simulink model "Control_test"  (R2014b)
settings: Solver=FixedStepDiscrete  StartTime=0.0  StopTime=Inf  FixedStep=0.001  RelTol=1e-3
PostLoadFcn:
  | , if any(exist('dsrtsu_mdlpostloadfcn', 'file') == [2, 3, 6]), try dsrtsu_mdlpostloadfcn('Execute', bdroot); catch fprintf('Error in PostLoadFcn (dsrtsu_mdlpostloadfcn) for model "%s":\n %s\n', bdroot, lasterr); end, end,
undefined symbols (not defined in the file or in its folder): dtLocal, slcm
libraries: rtican x163, simulink x14
(part 14 of 34)

== system Control_test/InputProcessing/RadarCanProcessing/ESR_Sim1 ==
  Bus Creator : BusCreator  Inputs=9
  ESR_Sim1 : rtican/RTICAN Receive (RX)   Reserved1=[]  Reserved2=[]  Reserved3=[]  Reserved4=[]  SfcnMessage=[]  Msg_Struct=[]  BoardTypeNo=[]  BoardNo=[]  ChannelNo=[]  Parameters=[]  DialogFcn=[]  UnitName=[]  Revision=[]  UnitValues=[]  DSProperties=struct('RTI',struct('Version',uint32(5),'BlockType',struct('isSLSource',uint8(1),'isSLSink',uint8(1),'isHWSource',uint8(0),'isHWSink',uint8(0),'isSetup',uint8(0),'isInline',uint8(1),'isNonInline',uint8(0),'isInterrupt',uint8(0),'isChannelwise',uint8(0)),'IOBoardType','RTICAN','UnitType','MESSAGE','Identifier','RX','DialogType','MSVC','BlockSet','RTICAN','SlaveProcessor','CAN'))  RTIBlockInterface=struct('OutputPortsWidth',int32([1 1 1 1 1 1 1 1 1]),'OutputPortsActive',[1 1 1 1 1 1 1 1 1],'OutputPortsName',{{'CAN_RX_SIM_RANGE_RATE','CAN_RX_SIM_RANGE_ACCEL','CAN_RX_SIM_RANGE','CAN_RX_SIM_LAT_RATE','CAN_RX_SIM_LAT_POS','CAN_RX_SIM_ANGLE','CAN_RX_SIM_FUNCTION','CAN_RX_SIM_STATUS','CAN_RX_SIM_TRACK_ID'}},'OutputPortsDataType',{{'SS_DOUBLE','SS_DOUBLE','SS_DOUBLE','SS_DOUBLE','SS_DOUBLE','SS_DOUBLE','SS_DOUBLE','SS_DOUBLE','SS_DOUBLE'}},'OutputPortsLabel',{{'CAN_RX_SIM_RANGE_RATE','CAN_RX_SIM_RANGE_ACCEL','CAN_RX_SIM_RANGE','CAN_RX_SIM_LAT_RATE','CAN_RX_SIM_LAT_POS','CAN_RX_SIM_ANGLE','CAN_RX_SIM_FUNCTION','CAN_RX_SIM_STATUS','CAN_RX_SIM_TRACK_ID'}},'OutputPortsLabelMode','ON','InputPortsWidth',int32(0),'InputPortsActive',0,'DialogFcn','rtican_message_interface_gui','BlockDisplay',{{'','center'}},'IconTransparency','on','ParameterTunableNames',{{}},'InitLevel',3,'BlockName',struct('Token',{{'ESR_Sim1'}}),'SampleTime',{{-1}},'TriggerPort',{{'none'}},'EnablePort',{{'none'}})  RTIBlockParameters=struct('BoardTypeNo',{{1,'OFF',[]}},'BoardNo',{{2,'ON',[1 16]}},'ChannelNo',{{2,'ON',[1 2]}},'Parameters',{{struct('DataFileSupport',struct('DataFileSelectedMaster',1,'DataFileSelectedLocal',1,'DataFileName','c:\users\mpc_car\documents\github\mpc-car\controller\dbcfiles\esr_dv3_64tgt.dbc|','DataFileDate',['26-Aug-2014 13:16:21'],'SelectedFile','..\..\dbcfiles\esr_dv3_64tgt.dbc','InterfaceFcn','rtican_dbc_file_parser'),'Options',struct('StatusSelected',0,'TimeSelected',0,'DeltaTimeSelected',0,'BytePortSelected',0,'MessageLengthSelected',0,'TriggerPort',struct('Selected',0,'TriggerType',0),'UserCoding',struct('Selected',0,'InterfaceFile','UserDecodingFile','FcnName','UserDecodeFcn','InportSelected',0,'InportWidth',1,'OutportSelected',0,'OutportWidth',1),'EnablePortSelected',0,'SignalOnPortnameSelected',1,'UseRXService',0),'Message',struct('MsgOnBlocknameSelected',1,'MsgName','ESR_Sim1','MsgIdFormat',0,'MsgId',1472,'MsgLength',8,'NumSignals',9,'SampleTime',-1,'Signal',struct('SgnName',{'CAN_RX_SIM_RANGE_RATE','CAN_RX_SIM_RANGE_ACCEL','CAN_RX_SIM_RANGE','CAN_RX_SIM_LAT_RATE','CAN_RX_SIM_LAT_POS','CAN_RX_SIM_ANGLE','CAN_RX_SIM_FUNCTION','CAN_RX_SIM_STATUS','CAN_RX_SIM_TRACK_ID'},'SgnStartBit',{8,16,24,32,40,48,56,59,61},'SgnLength',{8,8,8,8,8,8,3,2,2},'ByteLayout',{2,2,2,2,2,2,2,2,2},'Factor',{0.25,0.25,1,0.25,0.25,0.5,1,1,1},'Offset',{0,0,0,0,0,0,0,0,0},'SgnComment',{'','','','','','','','',''},'SgnUnit',{'m/s','m/s/s','m','m/s','m','deg','','',''},'Min',{-32,-32,0,-32,-32,-64,0,0,0},'Max',{31.75,31.75,0,31.75,31.75,63.5,0,0,0},'SgnType',{0,0,0,0,0,0,0,0,0},'SLDataType',{'SS_DOUBLE','SS_DOUBLE','SS_DOUBLE','SS_DOUBLE','SS_DOUBLE','SS_DOUBLE','SS_DOUBLE','SS_DOUBLE','SS_DOUBLE'},'DataType',{1,1,0,1,1,1,0,0,0},'ModeValue',{-1,-1,-1,-1,-1,-1,-1,-1,-1}),'MsgIdNumFormat',0,'MsgComment',{{''}}),'Version',1.2,'general',struct('isFromLib',0)),'OFF',[]}},'GroupId',{{struct('Group',{{'RTICAN'}},'No',4,'Behavior',{{'NAMECHANGE'}},'BlockType',{{'SINK'}},'NameChangeFlag',0),'OFF',[]}},'SFcnRTICANMessage',{{struct('MsgType','RX','SFcnPortType','Scalar','MsgName','ESR_Sim1','MsgIdFormat','STD','MsgId',1472,'MsgLength',8,'NumSignals',9,'SampleTime',-1,'Signal',struct('SgnName',{'CAN_RX_SIM_RANGE_RATE','CAN_RX_SIM_RANGE_ACCEL','CAN_RX_SIM_RANGE','CAN_RX_SIM_LAT_RATE','CAN_RX_SIM_LAT_POS','CAN_RX_SIM_ANGLE','CAN_RX_SIM_FUNCTION','CAN_RX_SIM_STATUS','CAN_RX_SIM_TRACK_ID'},'SgnStartBit',{8,16,24,32,40,48,56,59,61},'SgnLength',{8,8,8,8,8,8,3,2,2},'ByteLayout',{['motorola back.'],['motorola back.'],['motorola back.'],['motorola back.'],['motorola back.'],['motorola back.'],['motorola back.'],['motorola back.'],['motorola back.']},'Factor',{0.25,0.25,1,0.25,0.25,0.5,1,1,1},'Offset',{0,0,0,0,0,0,0,0,0},'SgnType',{'standard','standard','standard','standard','standard','standard','standard','standard','standard'},'SLDataType',{'SS_DOUBLE','SS_DOUBLE','SS_DOUBLE','SS_DOUBLE','SS_DOUBLE','SS_DOUBLE','SS_DOUBLE','SS_DOUBLE','SS_DOUBLE'},'DataType',{['signed int'],['signed int'],['unsigned int'],['signed int'],['signed int'],['signed int'],['unsigned int'],['unsigned int'],['unsigned int']},'ModeValue',{-1,-1,-1,-1,-1,-1,-1,-1,-1}),'StatusSelected','no','TimeSelected','no','DeltaTimeSelected','no','BytePortSelected','no','MessageLengthSelected','no','TriggerPort',struct('Selected','no','TriggerType',0),'UserCoding',struct('Selected','no','InterfaceFile','UserDecodingFile','FcnName','UserDecodeFcn','InportSelected','no','InportWidth',1,'OutportSelected','no','OutportWidth',1),'EnablePortSelected','no','UseRXService','no','BoardType','DS1','BoardNo',2,'ControllerNo',2),'OFF',[]}},'TLCFileName',{{'rtican_rx_message','OFF',[]}})  RTISFcnParameters=struct('SFcnRTICANMessage','struct','TLCFileName','char')  RTIBlockParaDefault=struct('BoardTypeNo',4302,'BoardNo',1,'ChannelNo',1,'Parameters',struct('DataFileSupport',struct('DataFileSelectedMaster',0,'DataFileSelectedLocal',0,'DataFileName','','DataFileDate','','SelectedFile',['<no file selected>']),'Options',struct('StatusSelected',1,'TimeSelected',1,'DeltaTimeSelected',1,'BytePortSelected',0,'MessageLengthSelected',0,'TriggerPort',struct('Selected',0,'TriggerType','rising'),'UserCoding',struct('Selected',0,'InterfaceFile','UserDecodingFile','FcnName','UserDecodeFcn','InportSelected',0,'InportWidth',1,'OutportSelected',0,'OutportWidth',1),'EnablePortSelected',0,'SignalOnPortnameSelected',1,'UseRXService',0),'Message',struct('MsgOnBlocknameSelected',0,'MsgName',['RX Message'],'MsgIdFormat',0,'MsgId',100,'MsgLength',8,'NumSignals',1,'SampleTime',-1,'Signal',struct('SgnName',['RX signal'],'SgnStartBit',0,'SgnLength',8,'SgnType',0,'ModeValue',-1,'DataType',0,'SLDataType','SS_DOUBLE','ByteLayout',0,'Factor',1,'Offset',0,'Min',0,'Max',255,'SgnComment',{{}},'SgnUnit',''),'MsgIdNumFormat',0,'MsgComment',{{''}}),'Version',1.2,'general',struct('isFromLib',1)),'GroupId',struct('Group',{{'RTICAN'}},'No',1,'Behavior',{{'NAMECHANGE'}},'BlockType',{{'SINK'}},'NameChangeFlag',0),'SFcnRTICANMessage',struct('MsgType','RX','MsgName',['RX Message'],'MsgIdFormat','STD','MsgId',100,'MsgLength',8,'NumSignals',1,'SampleTime',-1,'Signal',struct('SgnName',['RX signal'],'SgnStartBit',0,'SgnLength',8,'SgnType','standard','ModeValue',-1,'DataType',['unsigned int'],'ByteLayout',['little endian'],'SLDataType','SS_DOUBLE','Factor',1,'Offset',0),'StatusSelected','yes','TimeSelected','yes','DeltaTimeSelected','yes','BytePortSelected','no','MessageLengthSelected','no','EnablePortSelected','no','UserCoding',struct('Selected','no','InterfaceFile','UserDecodingFile','FcnName','UserDecodeFcn','InportSelected','no','InportWidth',1,'OutportSelected','no','OutportWidth',1),'TriggerPort',struct('Selected','no','TriggerType','rising'),'UseRXService','no','BoardType','DS4302','BoardNo',1,'ControllerNo',1,'SFcnPortType','Scalar'),'TLCFileName','rtican_rx_message')
      settings: AttributesFormatString=Group Id: RTICAN4\n
  ESR_Sim_1 : Outport
  wires:
  Bus Creator/1 -> ESR_Sim_1/1  "ESR_Sim1"
  ESR_Sim1/1 -> Bus Creator/1  "CAN_RX_SIM_RANGE_RATE"
  ESR_Sim1/2 -> Bus Creator/2  "CAN_RX_SIM_RANGE_ACCEL"
  ESR_Sim1/3 -> Bus Creator/3  "CAN_RX_SIM_RANGE"
  ESR_Sim1/4 -> Bus Creator/4  "CAN_RX_SIM_LAT_RATE"
  ESR_Sim1/5 -> Bus Creator/5  "CAN_RX_SIM_LAT_POS"
  ESR_Sim1/6 -> Bus Creator/6  "CAN_RX_SIM_ANGLE"
  ESR_Sim1/7 -> Bus Creator/7  "CAN_RX_SIM_FUNCTION"
  ESR_Sim1/8 -> Bus Creator/8  "CAN_RX_SIM_STATUS"
  ESR_Sim1/9 -> Bus Creator/9  "CAN_RX_SIM_TRACK_ID"

== system Control_test/InputProcessing/RadarCanProcessing/ESR_Status1 ==
  Bus Creator : BusCreator  Inputs=7
  ESR_Status1 : rtican/RTICAN Receive (RX)   Reserved1=[]  Reserved2=[]  Reserved3=[]  Reserved4=[]  SfcnMessage=[]  Msg_Struct=[]  BoardTypeNo=[]  BoardNo=[]  ChannelNo=[]  Parameters=[]  DialogFcn=[]  UnitName=[]  Revision=[]  UnitValues=[]  DSProperties=struct('RTI',struct('Version',uint32(5),'BlockType',struct('isSLSource',uint8(1),'isSLSink',uint8(1),'isHWSource',uint8(0),'isHWSink',uint8(0),'isSetup',uint8(0),'isInline',uint8(1),'isNonInline',uint8(0),'isInterrupt',uint8(0),'isChannelwise',uint8(0)),'IOBoardType','RTICAN','UnitType','MESSAGE','Identifier','RX','DialogType','MSVC','BlockSet','RTICAN','SlaveProcessor','CAN'))  RTIBlockInterface=struct('OutputPortsWidth',int32([1 1 1 1 1 1 1]),'OutputPortsActive',[1 1 1 1 1 1 1],'OutputPortsName',{{'CAN_TX_VEHICLE_SPEED_CALC','CAN_TX_YAW_RATE_CALC','CAN_TX_SCAN_INDEX','CAN_TX_RADIUS_CURVATURE_CALC','CAN_TX_COMM_ERROR','CAN_TX_DSP_TIMESTAMP','CAN_TX_ROLLING_COUNT_1'}},'OutputPortsDataType',{{'SS_DOUBLE','SS_DOUBLE','SS_DOUBLE','SS_DOUBLE','SS_DOUBLE','SS_DOUBLE','SS_DOUBLE'}},'OutputPortsLabel',{{'CAN_TX_VEHICLE_SPEED_CALC','CAN_TX_YAW_RATE_CALC','CAN_TX_SCAN_INDEX','CAN_TX_RADIUS_CURVATURE_CALC','CAN_TX_COMM_ERROR','CAN_TX_DSP_TIMESTAMP','CAN_TX_ROLLING_COUNT_1'}},'OutputPortsLabelMode','ON','InputPortsWidth',int32(0),'InputPortsActive',0,'DialogFcn','rtican_message_interface_gui','BlockDisplay',{{'','center'}},'IconTransparency','on','ParameterTunableNames',{{}},'InitLevel',3,'BlockName',struct('Token',{{'ESR_Status1'}}),'SampleTime',{{-1}},'TriggerPort',{{'none'}},'EnablePort',{{'none'}})  RTIBlockParameters=struct('BoardTypeNo',{{1,'OFF',[]}},'BoardNo',{{2,'ON',[1 16]}},'ChannelNo',{{2,'ON',[1 2]}},'Parameters',{{struct('DataFileSupport',struct('DataFileSelectedMaster',1,'DataFileSelectedLocal',1,'DataFileName',['c:\users\mpc\dropbox\hyundai car setup\esr_dv3_64tgt.dbc|'],'DataFileDate',['26-Aug-2014 13:16:21'],'SelectedFile','..\..\dbcfiles\esr_dv3_64tgt.dbc','InterfaceFcn','rtican_dbc_file_parser'),'Options',struct('StatusSelected',0,'TimeSelected',0,'DeltaTimeSelected',0,'BytePortSelected',0,'MessageLengthSelected',0,'TriggerPort',struct('Selected',0,'TriggerType',0),'UserCoding',struct('Selected',0,'InterfaceFile','UserDecodingFile','FcnName','UserDecodeFcn','InportSelected',0,'InportWidth',1,'OutportSelected',0,'OutportWidth',1),'EnablePortSelected',0,'SignalOnPortnameSelected',1,'UseRXService',0),'Message',struct('MsgOnBlocknameSelected',1,'MsgName','ESR_Status1','MsgIdFormat',0,'MsgId',1248,'MsgLength',8,'NumSignals',7,'SampleTime',-1,'Signal',struct('SgnName',{'CAN_TX_VEHICLE_SPEED_CALC','CAN_TX_YAW_RATE_CALC','CAN_TX_SCAN_INDEX','CAN_TX_RADIUS_CURVATURE_CALC','CAN_TX_COMM_ERROR','CAN_TX_DSP_TIMESTAMP','CAN_TX_ROLLING_COUNT_1'},'SgnStartBit',{0,12,24,40,54,55,62},'SgnLength',{11,12,16,14,1,7,2},'ByteLayout',{2,2,2,2,2,2,2},'Factor',{0.0625,0.0625,1,1,1,2,1},'Offset',{0,0,0,0,0,0,0},'SgnComment',{'','','','','','',''},'SgnUnit',{'m/s','deg/s','','m','','ms',''},'Min',{0,-128,0,-8192,0,0,0},'Max',{127.9375,127.9375,65535,8191,0,254,0},'SgnType',{0,0,0,0,0,0,0},'SLDataType',{'SS_DOUBLE','SS_DOUBLE','SS_DOUBLE','SS_DOUBLE','SS_DOUBLE','SS_DOUBLE','SS_DOUBLE'},'DataType',{0,1,0,1,0,0,0},'ModeValue',{-1,-1,-1,-1,-1,-1,-1}),'MsgIdNumFormat',0,'MsgComment',{{''}}),'Version',1.2,'general',struct('isFromLib',0)),'OFF',[]}},'GroupId',{{struct('Group',{{'RTICAN'}},'No',4,'Behavior',{{'NAMECHANGE'}},'BlockType',{{'SINK'}},'NameChangeFlag',0),'OFF',[]}},'SFcnRTICANMessage',{{struct('MsgType','RX','SFcnPortType','Scalar','MsgName','ESR_Status1','MsgIdFormat','STD','MsgId',1248,'MsgLength',8,'NumSignals',7,'SampleTime',-1,'Signal',struct('SgnName',{'CAN_TX_VEHICLE_SPEED_CALC','CAN_TX_YAW_RATE_CALC','CAN_TX_SCAN_INDEX','CAN_TX_RADIUS_CURVATURE_CALC','CAN_TX_COMM_ERROR','CAN_TX_DSP_TIMESTAMP','CAN_TX_ROLLING_COUNT_1'},'SgnStartBit',{0,12,24,40,54,55,62},'SgnLength',{11,12,16,14,1,7,2},'ByteLayout',{['motorola back.'],['motorola back.'],['motorola back.'],['motorola back.'],['motorola back.'],['motorola back.'],['motorola back.']},'Factor',{0.0625,0.0625,1,1,1,2,1},'Offset',{0,0,0,0,0,0,0},'SgnType',{'standard','standard','standard','standard','standard','standard','standard'},'SLDataType',{'SS_DOUBLE','SS_DOUBLE','SS_DOUBLE','SS_DOUBLE','SS_DOUBLE','SS_DOUBLE','SS_DOUBLE'},'DataType',{['unsigned int'],['signed int'],['unsigned int'],['signed int'],['unsigned int'],['unsigned int'],['unsigned int']},'ModeValue',{-1,-1,-1,-1,-1,-1,-1}),'StatusSelected','no','TimeSelected','no','DeltaTimeSelected','no','BytePortSelected','no','MessageLengthSelected','no','TriggerPort',struct('Selected','no','TriggerType',0),'UserCoding',struct('Selected','no','InterfaceFile','UserDecodingFile','FcnName','UserDecodeFcn','InportSelected','no','InportWidth',1,'OutportSelected','no','OutportWidth',1),'EnablePortSelected','no','UseRXService','no','BoardType','DS1','BoardNo',2,'ControllerNo',2),'OFF',[]}},'TLCFileName',{{'rtican_rx_message','OFF',[]}})  RTISFcnParameters=struct('SFcnRTICANMessage','struct','TLCFileName','char')  RTIBlockParaDefault=struct('BoardTypeNo',4302,'BoardNo',1,'ChannelNo',1,'Parameters',struct('DataFileSupport',struct('DataFileSelectedMaster',0,'DataFileSelectedLocal',0,'DataFileName','','DataFileDate','','SelectedFile',['<no file selected>']),'Options',struct('StatusSelected',1,'TimeSelected',1,'DeltaTimeSelected',1,'BytePortSelected',0,'MessageLengthSelected',0,'TriggerPort',struct('Selected',0,'TriggerType','rising'),'UserCoding',struct('Selected',0,'InterfaceFile','UserDecodingFile','FcnName','UserDecodeFcn','InportSelected',0,'InportWidth',1,'OutportSelected',0,'OutportWidth',1),'EnablePortSelected',0,'SignalOnPortnameSelected',1,'UseRXService',0),'Message',struct('MsgOnBlocknameSelected',0,'MsgName',['RX Message'],'MsgIdFormat',0,'MsgId',100,'MsgLength',8,'NumSignals',1,'SampleTime',-1,'Signal',struct('SgnName',['RX signal'],'SgnStartBit',0,'SgnLength',8,'SgnType',0,'ModeValue',-1,'DataType',0,'SLDataType','SS_DOUBLE','ByteLayout',0,'Factor',1,'Offset',0,'Min',0,'Max',255,'SgnComment',{{}},'SgnUnit',''),'MsgIdNumFormat',0,'MsgComment',{{''}}),'Version',1.2,'general',struct('isFromLib',1)),'GroupId',struct('Group',{{'RTICAN'}},'No',1,'Behavior',{{'NAMECHANGE'}},'BlockType',{{'SINK'}},'NameChangeFlag',0),'SFcnRTICANMessage',struct('MsgType','RX','MsgName',['RX Message'],'MsgIdFormat','STD','MsgId',100,'MsgLength',8,'NumSignals',1,'SampleTime',-1,'Signal',struct('SgnName',['RX signal'],'SgnStartBit',0,'SgnLength',8,'SgnType','standard','ModeValue',-1,'DataType',['unsigned int'],'ByteLayout',['little endian'],'SLDataType','SS_DOUBLE','Factor',1,'Offset',0),'StatusSelected','yes','TimeSelected','yes','DeltaTimeSelected','yes','BytePortSelected','no','MessageLengthSelected','no','EnablePortSelected','no','UserCoding',struct('Selected','no','InterfaceFile','UserDecodingFile','FcnName','UserDecodeFcn','InportSelected','no','InportWidth',1,'OutportSelected','no','OutportWidth',1),'TriggerPort',struct('Selected','no','TriggerType','rising'),'UseRXService','no','BoardType','DS4302','BoardNo',1,'ControllerNo',1,'SFcnPortType','Scalar'),'TLCFileName','rtican_rx_message')
      settings: AttributesFormatString=Group Id: RTICAN4\n
  ESR_Status_1 : Outport
  wires:
  Bus Creator/1 -> ESR_Status_1/1  "ESR_Status1"
  ESR_Status1/1 -> Bus Creator/1  "CAN_TX_VEHICLE_SPEED_CALC"
  ESR_Status1/2 -> Bus Creator/2  "CAN_TX_YAW_RATE_CALC"
  ESR_Status1/3 -> Bus Creator/3  "CAN_TX_SCAN_INDEX"
  ESR_Status1/4 -> Bus Creator/4  "CAN_TX_RADIUS_CURVATURE_CALC"
  ESR_Status1/5 -> Bus Creator/5  "CAN_TX_COMM_ERROR"
  ESR_Status1/6 -> Bus Creator/6  "CAN_TX_DSP_TIMESTAMP"
  ESR_Status1/7 -> Bus Creator/7  "CAN_TX_ROLLING_COUNT_1"

== system Control_test/InputProcessing/RadarCanProcessing/ESR_Status2 ==
  Bus Creator : BusCreator  Inputs=13
  ESR_Status2 : rtican/RTICAN Receive (RX)   Reserved1=[]  Reserved2=[]  Reserved3=[]  Reserved4=[]  SfcnMessage=[]  Msg_Struct=[]  BoardTypeNo=[]  BoardNo=[]  ChannelNo=[]  Parameters=[]  DialogFcn=[]  UnitName=[]  Revision=[]  UnitValues=[]  DSProperties=struct('RTI',struct('Version',uint32(5),'BlockType',struct('isSLSource',uint8(1),'isSLSink',uint8(1),'isHWSource',uint8(0),'isHWSink',uint8(0),'isSetup',uint8(0),'isInline',uint8(1),'isNonInline',uint8(0),'isInterrupt',uint8(0),'isChannelwise',uint8(0)),'IOBoardType','RTICAN','UnitType','MESSAGE','Identifier','RX','DialogType','MSVC','BlockSet','RTICAN','SlaveProcessor','CAN'))  RTIBlockInterface=struct('OutputPortsWidth',int32([1 1 1 1 1 1 1 1 1 1 1 1 1]),'OutputPortsActive',[1 1 1 1 1 1 1 1 1 1 1 1 1],'OutputPortsName',{{'CAN_TX_SW_VERSION_DSP','CAN_TX_YAW_RATE_BIAS','CAN_TX_GROUPING_MODE','CAN_TX_VEH_SPD_COMP_FACTOR','CAN_TX_TEMPERATURE','CAN_TX_STEERING_ANGLE_ACK','CAN_TX_RAW_DATA_MODE','CAN_TX_XCVR_OPERATIONAL','CAN_TX_INTERNAL_ERROR','CAN_TX_RANGE_PERF_ERROR','CAN_TX_OVERHEAT_ERROR','CAN_TX_ROLLING_COUNT_2','CAN_TX_MAXIMUM_TRACKS_ACK'}},'OutputPortsDataType',{{'SS_DOUBLE','SS_DOUBLE','SS_DOUBLE','SS_DOUBLE','SS_DOUBLE','SS_DOUBLE','SS_DOUBLE','SS_DOUBLE','SS_DOUBLE','SS_DOUBLE','SS_DOUBLE','SS_DOUBLE','SS_DOUBLE'}},'OutputPortsLabel',{{'CAN_TX_SW_VERSION_DSP','CAN_TX_YAW_RATE_BIAS','CAN_TX_GROUPING_MODE','CAN_TX_VEH_SPD_COMP_FACTOR','CAN_TX_TEMPERATURE','CAN_TX_STEERING_ANGLE_ACK','CAN_TX_RAW_DATA_MODE','CAN_TX_XCVR_OPERATIONAL','CAN_TX_INTERNAL_ERROR','CAN_TX_RANGE_PERF_ERROR','CAN_TX_OVERHEAT_ERROR','CAN_TX_ROLLING_COUNT_2','CAN_TX_MAXIMUM_TRACKS_ACK'}},'OutputPortsLabelMode','ON','InputPortsWidth',int32(0),'InputPortsActive',0,'DialogFcn','rtican_message_interface_gui','BlockDisplay',{{'','center'}},'IconTransparency','on','ParameterTunableNames',{{}},'InitLevel',3,'BlockName',struct('Token',{{'ESR_Status2'}}),'SampleTime',{{-1}},'TriggerPort',{{'none'}},'EnablePort',{{'none'}})  RTIBlockParameters=struct('BoardTypeNo',{{1,'OFF',[]}},'BoardNo',{{2,'ON',[1 16]}},'ChannelNo',{{2,'ON',[1 2]}},'Parameters',{{struct('DataFileSupport',struct('DataFileSelectedMaster',1,'DataFileSelectedLocal',1,'DataFileName',['c:\users\mpc\dropbox\hyundai car setup\esr_dv3_64tgt.dbc|'],'DataFileDate',['26-Aug-2014 13:16:21'],'SelectedFile','..\..\dbcfiles\esr_dv3_64tgt.dbc','InterfaceFcn','rtican_dbc_file_parser'),'Options',struct('StatusSelected',0,'TimeSelected',0,'DeltaTimeSelected',0,'BytePortSelected',0,'MessageLengthSelected',0,'TriggerPort',struct('Selected',0,'TriggerType',0),'UserCoding',struct('Selected',0,'InterfaceFile','UserDecodingFile','FcnName','UserDecodeFcn','InportSelected',0,'InportWidth',1,'OutportSelected',0,'OutportWidth',1),'EnablePortSelected',0,'SignalOnPortnameSelected',1,'UseRXService',0),'Message',struct('MsgOnBlocknameSelected',1,'MsgName','ESR_Status2','MsgIdFormat',0,'MsgId',1249,'MsgLength',8,'NumSignals',13,'SampleTime',-1,'Signal',struct('SgnName',{'CAN_TX_SW_VERSION_DSP','CAN_TX_YAW_RATE_BIAS','CAN_TX_GROUPING_MODE','CAN_TX_VEH_SPD_COMP_FACTOR','CAN_TX_TEMPERATURE','CAN_TX_STEERING_ANGLE_ACK','CAN_TX_RAW_DATA_MODE','CAN_TX_XCVR_OPERATIONAL','CAN_TX_INTERNAL_ERROR','CAN_TX_RANGE_PERF_ERROR','CAN_TX_OVERHEAT_ERROR','CAN_TX_ROLLING_COUNT_2','CAN_TX_MAXIMUM_TRACKS_ACK'},'SgnStartBit',{0,16,24,26,32,40,51,52,53,54,55,56,58},'SgnLength',{16,8,2,6,8,11,1,1,1,1,1,2,6},'ByteLayout',{2,2,2,2,2,2,2,2,2,2,2,2,2},'Factor',{1,0.125,1,0.001953125,1,1,1,1,1,1,1,1,1},'Offset',{0,0,0,1,0,0,0,0,0,0,0,0,1},'SgnComment',{'','','','','','','','','','','','',''},'SgnUnit',{'','','','','degC','deg','','','','','','',''},'Min',{0,-16,0,0.9375,-128,0,0,0,0,0,0,0,1},'Max',{0,15.875,0,1.060546875,127,2047,0,0,0,0,0,0,64},'SgnType',{0,0,0,0,0,0,0,0,0,0,0,0,0},'SLDataType',{'SS_DOUBLE','SS_DOUBLE','SS_DOUBLE','SS_DOUBLE','SS_DOUBLE','SS_DOUBLE','SS_DOUBLE','SS_DOUBLE','SS_DOUBLE','SS_DOUBLE','SS_DOUBLE','SS_DOUBLE','SS_DOUBLE'},'DataType',{0,1,0,1,1,0,0,0,0,0,0,0,0},'ModeValue',{-1,-1,-1,-1,-1,-1,-1,-1,-1,-1,-1,-1,-1}),'MsgIdNumFormat',0,'MsgComment',{{''}}),'Version',1.2,'general',struct('isFromLib',0)),'OFF',[]}},'GroupId',{{struct('Group',{{'RTICAN'}},'No',4,'Behavior',{{'NAMECHANGE'}},'BlockType',{{'SINK'}},'NameChangeFlag',0),'OFF',[]}},'SFcnRTICANMessage',{{struct('MsgType','RX','SFcnPortType','Scalar','MsgName','ESR_Status2','MsgIdFormat','STD','MsgId',1249,'MsgLength',8,'NumSignals',13,'SampleTime',-1,'Signal',struct('SgnName',{'CAN_TX_SW_VERSION_DSP','CAN_TX_YAW_RATE_BIAS','CAN_TX_GROUPING_MODE','CAN_TX_VEH_SPD_COMP_FACTOR','CAN_TX_TEMPERATURE','CAN_TX_STEERING_ANGLE_ACK','CAN_TX_RAW_DATA_MODE','CAN_TX_XCVR_OPERATIONAL','CAN_TX_INTERNAL_ERROR','CAN_TX_RANGE_PERF_ERROR','CAN_TX_OVERHEAT_ERROR','CAN_TX_ROLLING_COUNT_2','CAN_TX_MAXIMUM_TRACKS_ACK'},'SgnStartBit',{0,16,24,26,32,40,51,52,53,54,55,56,58},'SgnLength',{16,8,2,6,8,11,1,1,1,1,1,2,6},'ByteLayout',{['motorola back.'],['motorola back.'],['motorola back.'],['motorola back.'],['motorola back.'],['motorola back.'],['motorola back.'],['motorola back.'],['motorola back.'],['motorola back.'],['motorola back.'],['motorola back.'],['motorola back.']},'Factor',{1,0.125,1,0.001953125,1,1,1,1,1,1,1,1,1},'Offset',{0,0,0,1,0,0,0,0,0,0,0,0,1},'SgnType',{'standard','standard','standard','standard','standard','standard','standard','standard','standard','standard','standard','standard','standard'},'SLDataType',{'SS_DOUBLE','SS_DOUBLE','SS_DOUBLE','SS_DOUBLE','SS_DOUBLE','SS_DOUBLE','SS_DOUBLE','SS_DOUBLE','SS_DOUBLE','SS_DOUBLE','SS_DOUBLE','SS_DOUBLE','SS_DOUBLE'},'DataType',{['unsigned int'],['signed int'],['unsigned int'],['signed int'],['signed int'],['unsigned int'],['unsigned int'],['unsigned int'],['unsigned int'],['unsigned int'],['unsigned int'],['unsigned int'],['unsigned int']},'ModeValue',{-1,-1,-1,-1,-1,-1,-1,-1,-1,-1,-1,-1,-1}),'StatusSelected','no','TimeSelected','no','DeltaTimeSelected','no','BytePortSelected','no','MessageLengthSelected','no','TriggerPort',struct('Selected','no','TriggerType',0),'UserCoding',struct('Selected','no','InterfaceFile','UserDecodingFile','FcnName','UserDecodeFcn','InportSelected','no','InportWidth',1,'OutportSelected','no','OutportWidth',1),'EnablePortSelected','no','UseRXService','no','BoardType','DS1','BoardNo',2,'ControllerNo',2),'OFF',[]}},'TLCFileName',{{'rtican_rx_message','OFF',[]}})  RTISFcnParameters=struct('SFcnRTICANMessage','struct','TLCFileName','char')  RTIBlockParaDefault=struct('BoardTypeNo',4302,'BoardNo',1,'ChannelNo',1,'Parameters',struct('DataFileSupport',struct('DataFileSelectedMaster',0,'DataFileSelectedLocal',0,'DataFileName','','DataFileDate','','SelectedFile',['<no file selected>']),'Options',struct('StatusSelected',1,'TimeSelected',1,'DeltaTimeSelected',1,'BytePortSelected',0,'MessageLengthSelected',0,'TriggerPort',struct('Selected',0,'TriggerType','rising'),'UserCoding',struct('Selected',0,'InterfaceFile','UserDecodingFile','FcnName','UserDecodeFcn','InportSelected',0,'InportWidth',1,'OutportSelected',0,'OutportWidth',1),'EnablePortSelected',0,'SignalOnPortnameSelected',1,'UseRXService',0),'Message',struct('MsgOnBlocknameSelected',0,'MsgName',['RX Message'],'MsgIdFormat',0,'MsgId',100,'MsgLength',8,'NumSignals',1,'SampleTime',-1,'Signal',struct('SgnName',['RX signal'],'SgnStartBit',0,'SgnLength',8,'SgnType',0,'ModeValue',-1,'DataType',0,'SLDataType','SS_DOUBLE','ByteLayout',0,'Factor',1,'Offset',0,'Min',0,'Max',255,'SgnComment',{{}},'SgnUnit',''),'MsgIdNumFormat',0,'MsgComment',{{''}}),'Version',1.2,'general',struct('isFromLib',1)),'GroupId',struct('Group',{{'RTICAN'}},'No',1,'Behavior',{{'NAMECHANGE'}},'BlockType',{{'SINK'}},'NameChangeFlag',0),'SFcnRTICANMessage',struct('MsgType','RX','MsgName',['RX Message'],'MsgIdFormat','STD','MsgId',100,'MsgLength',8,'NumSignals',1,'SampleTime',-1,'Signal',struct('SgnName',['RX signal'],'SgnStartBit',0,'SgnLength',8,'SgnType','standard','ModeValue',-1,'DataType',['unsigned int'],'ByteLayout',['little endian'],'SLDataType','SS_DOUBLE','Factor',1,'Offset',0),'StatusSelected','yes','TimeSelected','yes','DeltaTimeSelected','yes','BytePortSelected','no','MessageLengthSelected','no','EnablePortSelected','no','UserCoding',struct('Selected','no','InterfaceFile','UserDecodingFile','FcnName','UserDecodeFcn','InportSelected','no','InportWidth',1,'OutportSelected','no','OutportWidth',1),'TriggerPort',struct('Selected','no','TriggerType','rising'),'UseRXService','no','BoardType','DS4302','BoardNo',1,'ControllerNo',1,'SFcnPortType','Scalar'),'TLCFileName','rtican_rx_message')
      settings: AttributesFormatString=Group Id: RTICAN4\n
  ESR_Status2_1 : Outport
  wires:
  Bus Creator/1 -> ESR_Status2_1/1  "ESR_Status21"
  ESR_Status2/1 -> Bus Creator/1  "CAN_TX_SW_VERSION_DSP"
  ESR_Status2/2 -> Bus Creator/2  "CAN_TX_YAW_RATE_BIAS"
  ESR_Status2/3 -> Bus Creator/3  "CAN_TX_GROUPING_MODE"
  ESR_Status2/4 -> Bus Creator/4  "CAN_TX_VEH_SPD_COMP_FACTOR"
  ESR_Status2/5 -> Bus Creator/5  "CAN_TX_TEMPERATURE"
  ESR_Status2/6 -> Bus Creator/6  "CAN_TX_STEERING_ANGLE_ACK"
  ESR_Status2/7 -> Bus Creator/7  "CAN_TX_RAW_DATA_MODE"
  ESR_Status2/8 -> Bus Creator/8  "CAN_TX_XCVR_OPERATIONAL"
  ESR_Status2/9 -> Bus Creator/9  "CAN_TX_INTERNAL_ERROR"
  ESR_Status2/10 -> Bus Creator/10  "CAN_TX_RANGE_PERF_ERROR"
  ESR_Status2/11 -> Bus Creator/11  "CAN_TX_OVERHEAT_ERROR"
  ESR_Status2/12 -> Bus Creator/12  "CAN_TX_ROLLING_COUNT_2"
  ESR_Status2/13 -> Bus Creator/13  "CAN_TX_MAXIMUM_TRACKS_ACK"

== system Control_test/InputProcessing/RadarCanProcessing/ESR_Status3 ==
  Bus Creator : BusCreator  Inputs=5
  ESR_Status3 : rtican/RTICAN Receive (RX)   Reserved1=[]  Reserved2=[]  Reserved3=[]  Reserved4=[]  SfcnMessage=[]  Msg_Struct=[]  BoardTypeNo=[]  BoardNo=[]  ChannelNo=[]  Parameters=[]  DialogFcn=[]  UnitName=[]  Revision=[]  UnitValues=[]  DSProperties=struct('RTI',struct('Version',uint32(5),'BlockType',struct('isSLSource',uint8(1),'isSLSink',uint8(1),'isHWSource',uint8(0),'isHWSink',uint8(0),'isSetup',uint8(0),'isInline',uint8(1),'isNonInline',uint8(0),'isInterrupt',uint8(0),'isChannelwise',uint8(0)),'IOBoardType','RTICAN','UnitType','MESSAGE','Identifier','RX','DialogType','MSVC','BlockSet','RTICAN','SlaveProcessor','CAN'))  RTIBlockInterface=struct('OutputPortsWidth',int32([1 1 1 1 1]),'OutputPortsActive',[1 1 1 1 1],'OutputPortsName',{{'CAN_TX_SW_VERSION_PLD','CAN_TX_SERIAL_NUM','CAN_TX_SW_VERSION_HOST','CAN_TX_HW_VERSION','CAN_TX_INTERFACE_VERSION'}},'OutputPortsDataType',{{'SS_DOUBLE','SS_DOUBLE','SS_DOUBLE','SS_DOUBLE','SS_DOUBLE'}},'OutputPortsLabel',{{'CAN_TX_SW_VERSION_PLD','CAN_TX_SERIAL_NUM','CAN_TX_SW_VERSION_HOST','CAN_TX_HW_VERSION','CAN_TX_INTERFACE_VERSION'}},'OutputPortsLabelMode','ON','InputPortsWidth',int32(0),'InputPortsActive',0,'DialogFcn','rtican_message_interface_gui','BlockDisplay',{{'','center'}},'IconTransparency','on','ParameterTunableNames',{{}},'InitLevel',3,'BlockName',struct('Token',{{'ESR_Status3'}}),'SampleTime',{{-1}},'TriggerPort',{{'none'}},'EnablePort',{{'none'}})  RTIBlockParameters=struct('BoardTypeNo',{{1,'OFF',[]}},'BoardNo',{{2,'ON',[1 16]}},'ChannelNo',{{2,'ON',[1 2]}},'Parameters',{{struct('DataFileSupport',struct('DataFileSelectedMaster',1,'DataFileSelectedLocal',1,'DataFileName',['c:\users\mpc\dropbox\hyundai car setup\esr_dv3_64tgt.dbc|'],'DataFileDate',['26-Aug-2014 13:16:21'],'SelectedFile','..\..\dbcfiles\esr_dv3_64tgt.dbc','InterfaceFcn','rtican_dbc_file_parser'),'Options',struct('StatusSelected',0,'TimeSelected',0,'DeltaTimeSelected',0,'BytePortSelected',0,'MessageLengthSelected',0,'TriggerPort',struct('Selected',0,'TriggerType',0),'UserCoding',struct('Selected',0,'InterfaceFile','UserDecodingFile','FcnName','UserDecodeFcn','InportSelected',0,'InportWidth',1,'OutportSelected',0,'OutportWidth',1),'EnablePortSelected',0,'SignalOnPortnameSelected',1,'UseRXService',0),'Message',struct('MsgOnBlocknameSelected',1,'MsgName','ESR_Status3','MsgIdFormat',0,'MsgId',1250,'MsgLength',8,'NumSignals',5,'SampleTime',-1,'Signal',struct('SgnName',{'CAN_TX_SW_VERSION_PLD','CAN_TX_SERIAL_NUM','CAN_TX_SW_VERSION_HOST','CAN_TX_HW_VERSION','CAN_TX_INTERFACE_VERSION'},'SgnStartBit',{0,8,32,56,60},'SgnLength',{8,24,24,4,4},'ByteLayout',{2,2,2,2,2},'Factor',{1,1,1,1,1},'Offset',{0,0,0,0,0},'SgnComment',{'','','','',''},'SgnUnit',{'','','','',''},'Min',{0,0,0,0,0},'Max',{0,0,0,0,0},'SgnType',{0,0,0,0,0},'SLDataType',{'SS_DOUBLE','SS_DOUBLE','SS_DOUBLE','SS_DOUBLE','SS_DOUBLE'},'DataType',{0,0,0,0,0},'ModeValue',{-1,-1,-1,-1,-1}),'MsgIdNumFormat',0,'MsgComment',{{''}}),'Version',1.2,'general',struct('isFromLib',0)),'OFF',[]}},'GroupId',{{struct('Group',{{'RTICAN'}},'No',4,'Behavior',{{'NAMECHANGE'}},'BlockType',{{'SINK'}},'NameChangeFlag',0),'OFF',[]}},'SFcnRTICANMessage',{{struct('MsgType','RX','SFcnPortType','Scalar','MsgName','ESR_Status3','MsgIdFormat','STD','MsgId',1250,'MsgLength',8,'NumSignals',5,'SampleTime',-1,'Signal',struct('SgnName',{'CAN_TX_SW_VERSION_PLD','CAN_TX_SERIAL_NUM','CAN_TX_SW_VERSION_HOST','CAN_TX_HW_VERSION','CAN_TX_INTERFACE_VERSION'},'SgnStartBit',{0,8,32,56,60},'SgnLength',{8,24,24,4,4},'ByteLayout',{['motorola back.'],['motorola back.'],['motorola back.'],['motorola back.'],['motorola back.']},'Factor',{1,1,1,1,1},'Offset',{0,0,0,0,0},'SgnType',{'standard','standard','standard','standard','standard'},'SLDataType',{'SS_DOUBLE','SS_DOUBLE','SS_DOUBLE','SS_DOUBLE','SS_DOUBLE'},'DataType',{['unsigned int'],['unsigned int'],['unsigned int'],['unsigned int'],['unsigned int']},'ModeValue',{-1,-1,-1,-1,-1}),'StatusSelected','no','TimeSelected','no','DeltaTimeSelected','no','BytePortSelected','no','MessageLengthSelected','no','TriggerPort',struct('Selected','no','TriggerType',0),'UserCoding',struct('Selected','no','InterfaceFile','UserDecodingFile','FcnName','UserDecodeFcn','InportSelected','no','InportWidth',1,'OutportSelected','no','OutportWidth',1),'EnablePortSelected','no','UseRXService','no','BoardType','DS1','BoardNo',2,'ControllerNo',2),'OFF',[]}},'TLCFileName',{{'rtican_rx_message','OFF',[]}})  RTISFcnParameters=struct('SFcnRTICANMessage','struct','TLCFileName','char')  RTIBlockParaDefault=struct('BoardTypeNo',4302,'BoardNo',1,'ChannelNo',1,'Parameters',struct('DataFileSupport',struct('DataFileSelectedMaster',0,'DataFileSelectedLocal',0,'DataFileName','','DataFileDate','','SelectedFile',['<no file selected>']),'Options',struct('StatusSelected',1,'TimeSelected',1,'DeltaTimeSelected',1,'BytePortSelected',0,'MessageLengthSelected',0,'TriggerPort',struct('Selected',0,'TriggerType','rising'),'UserCoding',struct('Selected',0,'InterfaceFile','UserDecodingFile','FcnName','UserDecodeFcn','InportSelected',0,'InportWidth',1,'OutportSelected',0,'OutportWidth',1),'EnablePortSelected',0,'SignalOnPortnameSelected',1,'UseRXService',0),'Message',struct('MsgOnBlocknameSelected',0,'MsgName',['RX Message'],'MsgIdFormat',0,'MsgId',100,'MsgLength',8,'NumSignals',1,'SampleTime',-1,'Signal',struct('SgnName',['RX signal'],'SgnStartBit',0,'SgnLength',8,'SgnType',0,'ModeValue',-1,'DataType',0,'SLDataType','SS_DOUBLE','ByteLayout',0,'Factor',1,'Offset',0,'Min',0,'Max',255,'SgnComment',{{}},'SgnUnit',''),'MsgIdNumFormat',0,'MsgComment',{{''}}),'Version',1.2,'general',struct('isFromLib',1)),'GroupId',struct('Group',{{'RTICAN'}},'No',1,'Behavior',{{'NAMECHANGE'}},'BlockType',{{'SINK'}},'NameChangeFlag',0),'SFcnRTICANMessage',struct('MsgType','RX','MsgName',['RX Message'],'MsgIdFormat','STD','MsgId',100,'MsgLength',8,'NumSignals',1,'SampleTime',-1,'Signal',struct('SgnName',['RX signal'],'SgnStartBit',0,'SgnLength',8,'SgnType','standard','ModeValue',-1,'DataType',['unsigned int'],'ByteLayout',['little endian'],'SLDataType','SS_DOUBLE','Factor',1,'Offset',0),'StatusSelected','yes','TimeSelected','yes','DeltaTimeSelected','yes','BytePortSelected','no','MessageLengthSelected','no','EnablePortSelected','no','UserCoding',struct('Selected','no','InterfaceFile','UserDecodingFile','FcnName','UserDecodeFcn','InportSelected','no','InportWidth',1,'OutportSelected','no','OutportWidth',1),'TriggerPort',struct('Selected','no','TriggerType','rising'),'UseRXService','no','BoardType','DS4302','BoardNo',1,'ControllerNo',1,'SFcnPortType','Scalar'),'TLCFileName','rtican_rx_message')
      settings: AttributesFormatString=Group Id: RTICAN4\n
  ESR_Status3_1 : Outport
  wires:
  Bus Creator/1 -> ESR_Status3_1/1  "ESR_Status3"
  ESR_Status3/1 -> Bus Creator/1  "CAN_TX_SW_VERSION_PLD"
  ESR_Status3/2 -> Bus Creator/2  "CAN_TX_SERIAL_NUM"
  ESR_Status3/3 -> Bus Creator/3  "CAN_TX_SW_VERSION_HOST"
  ESR_Status3/4 -> Bus Creator/4  "CAN_TX_HW_VERSION"
  ESR_Status3/5 -> Bus Creator/5  "CAN_TX_INTERFACE_VERSION"

== system Control_test/InputProcessing/RadarCanProcessing/ESR_Status4 ==
  Bus Creator : BusCreator  Inputs=13
  ESR_Status4 : rtican/RTICAN Receive (RX)   Reserved1=[]  Reserved2=[]  Reserved3=[]  Reserved4=[]  SfcnMessage=[]  Msg_Struct=[]  BoardTypeNo=[]  BoardNo=[]  ChannelNo=[]  Parameters=[]  DialogFcn=[]  UnitName=[]  Revision=[]  UnitValues=[]  DSProperties=struct('RTI',struct('Version',uint32(5),'BlockType',struct('isSLSource',uint8(1),'isSLSink',uint8(1),'isHWSource',uint8(0),'isHWSink',uint8(0),'isSetup',uint8(0),'isInline',uint8(1),'isNonInline',uint8(0),'isInterrupt',uint8(0),'isChannelwise',uint8(0)),'IOBoardType','RTICAN','UnitType','MESSAGE','Identifier','RX','DialogType','MSVC','BlockSet','RTICAN','SlaveProcessor','CAN'))  RTIBlockInterface=struct('OutputPortsWidth',int32([1 1 1 1 1 1 1 1 1 1 1 1 1]),'OutputPortsActive',[1 1 1 1 1 1 1 1 1 1 1 1 1],'OutputPortsName',{{'CAN_TX_PATH_ID_ACC_STAT','CAN_TX_AUTO_ALIGN_ANGLE','CAN_TX_PATH_ID_FCW_STAT','CAN_TX_PATH_ID_FCW_MOVE','CAN_TX_PATH_ID_CMBB_STAT','CAN_TX_PATH_ID_CMBB_MOVE','CAN_TX_PATH_ID_ACC','CAN_TX_ROLLING_COUNT_3','CAN_TX_MR_LR_MODE','CAN_TX_PARTIAL_BLOCKAGE','CAN_TX_SIDELOBE_BLOCKAGE','CAN_TX_LR_ONLY_GRATING_LOBE_DET','CAN_TX_TRUCK_TARGET_DET'}},'OutputPortsDataType',{{'SS_DOUBLE','SS_DOUBLE','SS_DOUBLE','SS_DOUBLE','SS_DOUBLE','SS_DOUBLE','SS_DOUBLE','SS_DOUBLE','SS_DOUBLE','SS_DOUBLE','SS_DOUBLE','SS_DOUBLE','SS_DOUBLE'}},'OutputPortsLabel',{{'CAN_TX_PATH_ID_ACC_STAT','CAN_TX_AUTO_ALIGN_ANGLE','CAN_TX_PATH_ID_FCW_STAT','CAN_TX_PATH_ID_FCW_MOVE','CAN_TX_PATH_ID_CMBB_STAT','CAN_TX_PATH_ID_CMBB_MOVE','CAN_TX_PATH_ID_ACC','CAN_TX_ROLLING_COUNT_3','CAN_TX_MR_LR_MODE','CAN_TX_PARTIAL_BLOCKAGE','CAN_TX_SIDELOBE_BLOCKAGE','CAN_TX_LR_ONLY_GRATING_LOBE_DET','CAN_TX_TRUCK_TARGET_DET'}},'OutputPortsLabelMode','ON','InputPortsWidth',int32(0),'InputPortsActive',0,'DialogFcn','rtican_message_interface_gui','BlockDisplay',{{'','center'}},'IconTransparency','on','ParameterTunableNames',{{}},'InitLevel',3,'BlockName',struct('Token',{{'ESR_Status4'}}),'SampleTime',{{-1}},'TriggerPort',{{'none'}},'EnablePort',{{'none'}})  RTIBlockParameters=struct('BoardTypeNo',{{1,'OFF',[]}},'BoardNo',{{2,'ON',[1 16]}},'ChannelNo',{{2,'ON',[1 2]}},'Parameters',{{struct('DataFileSupport',struct('DataFileSelectedMaster',1,'DataFileSelectedLocal',1,'DataFileName','c:\users\mpc_car\documents\github\mpc-car\controller\dbcfiles\esr_dv3_64tgt.dbc|','DataFileDate',['26-Aug-2014 13:16:21'],'SelectedFile','..\..\dbcfiles\esr_dv3_64tgt.dbc','InterfaceFcn','rtican_dbc_file_parser'),'Options',struct('StatusSelected',0,'TimeSelected',0,'DeltaTimeSelected',0,'BytePortSelected',0,'MessageLengthSelected',0,'TriggerPort',struct('Selected',0,'TriggerType',0),'UserCoding',struct('Selected',0,'InterfaceFile','UserDecodingFile','FcnName','UserDecodeFcn','InportSelected',0,'InportWidth',1,'OutportSelected',0,'OutportWidth',1),'EnablePortSelected',0,'SignalOnPortnameSelected',1,'UseRXService',0),'Message',struct('MsgOnBlocknameSelected',1,'MsgName','ESR_Status4','MsgIdFormat',0,'MsgId',1251,'MsgLength',8,'NumSignals',13,'SampleTime',-1,'Signal',struct('SgnName',{'CAN_TX_PATH_ID_ACC_STAT','CAN_TX_AUTO_ALIGN_ANGLE','CAN_TX_PATH_ID_FCW_STAT','CAN_TX_PATH_ID_FCW_MOVE','CAN_TX_PATH_ID_CMBB_STAT','CAN_TX_PATH_ID_CMBB_MOVE','CAN_TX_PATH_ID_ACC','CAN_TX_ROLLING_COUNT_3','CAN_TX_MR_LR_MODE','CAN_TX_PARTIAL_BLOCKAGE','CAN_TX_SIDELOBE_BLOCKAGE','CAN_TX_LR_ONLY_GRATING_LOBE_DET','CAN_TX_TRUCK_TARGET_DET'},'SgnStartBit',{0,8,16,24,32,40,48,56,58,60,61,62,63},'SgnLength',{8,8,8,8,8,8,8,2,2,1,1,1,1},'ByteLayout',{2,2,2,2,2,2,2,2,2,2,2,2,2},'Factor',{1,0.0625,1,1,1,1,1,1,1,1,1,1,1},'Offset',{0,0,0,0,0,0,0,0,0,0,0,0,0},'SgnComment',{'','','','','','','','','','','','',''},'SgnUnit',{'','','','','','','','','','','','',''},'Min',{0,-8,0,0,0,0,0,0,0,0,0,0,0},'Max',{0,7.9375,0,0,0,0,0,0,3,0,0,0,0},'SgnType',{0,0,0,0,0,0,0,0,0,0,0,0,0},'SLDataType',{'SS_DOUBLE','SS_DOUBLE','SS_DOUBLE','SS_DOUBLE','SS_DOUBLE','SS_DOUBLE','SS_DOUBLE','SS_DOUBLE','SS_DOUBLE','SS_DOUBLE','SS_DOUBLE','SS_DOUBLE','SS_DOUBLE'},'DataType',{0,1,0,0,0,0,0,0,0,0,0,0,0},'ModeValue',{-1,-1,-1,-1,-1,-1,-1,-1,-1,-1,-1,-1,-1}),'MsgIdNumFormat',0,'MsgComment',{{''}}),'Version',1.2,'general',struct('isFromLib',0)),'OFF',[]}},'GroupId',{{struct('Group',{{'RTICAN'}},'No',4,'Behavior',{{'NAMECHANGE'}},'BlockType',{{'SINK'}},'NameChangeFlag',0),'OFF',[]}},'SFcnRTICANMessage',{{struct('MsgType','RX','SFcnPortType','Scalar','MsgName','ESR_Status4','MsgIdFormat','STD','MsgId',1251,'MsgLength',8,'NumSignals',13,'SampleTime',-1,'Signal',struct('SgnName',{'CAN_TX_PATH_ID_ACC_STAT','CAN_TX_AUTO_ALIGN_ANGLE','CAN_TX_PATH_ID_FCW_STAT','CAN_TX_PATH_ID_FCW_MOVE','CAN_TX_PATH_ID_CMBB_STAT','CAN_TX_PATH_ID_CMBB_MOVE','CAN_TX_PATH_ID_ACC','CAN_TX_ROLLING_COUNT_3','CAN_TX_MR_LR_MODE','CAN_TX_PARTIAL_BLOCKAGE','CAN_TX_SIDELOBE_BLOCKAGE','CAN_TX_LR_ONLY_GRATING_LOBE_DET','CAN_TX_TRUCK_TARGET_DET'},'SgnStartBit',{0,8,16,24,32,40,48,56,58,60,61,62,63},'SgnLength',{8,8,8,8,8,8,8,2,2,1,1,1,1},'ByteLayout',{['motorola back.'],['motorola back.'],['motorola back.'],['motorola back.'],['motorola back.'],['motorola back.'],['motorola back.'],['motorola back.'],['motorola back.'],['motorola back.'],['motorola back.'],['motorola back.'],['motorola back.']},'Factor',{1,0.0625,1,1,1,1,1,1,1,1,1,1,1},'Offset',{0,0,0,0,0,0,0,0,0,0,0,0,0},'SgnType',{'standard','standard','standard','standard','standard','standard','standard','standard','standard','standard','standard','standard','standard'},'SLDataType',{'SS_DOUBLE','SS_DOUBLE','SS_DOUBLE','SS_DOUBLE','SS_DOUBLE','SS_DOUBLE','SS_DOUBLE','SS_DOUBLE','SS_DOUBLE','SS_DOUBLE','SS_DOUBLE','SS_DOUBLE','SS_DOUBLE'},'DataType',{['unsigned int'],['signed int'],['unsigned int'],['unsigned int'],['unsigned int'],['unsigned int'],['unsigned int'],['unsigned int'],['unsigned int'],['unsigned int'],['unsigned int'],['unsigned int'],['unsigned int']},'ModeValue',{-1,-1,-1,-1,-1,-1,-1,-1,-1,-1,-1,-1,-1}),'StatusSelected','no','TimeSelected','no','DeltaTimeSelected','no','BytePortSelected','no','MessageLengthSelected','no','TriggerPort',struct('Selected','no','TriggerType',0),'UserCoding',struct('Selected','no','InterfaceFile','UserDecodingFile','FcnName','UserDecodeFcn','InportSelected','no','InportWidth',1,'OutportSelected','no','OutportWidth',1),'EnablePortSelected','no','UseRXService','no','BoardType','DS1','BoardNo',2,'ControllerNo',2),'OFF',[]}},'TLCFileName',{{'rtican_rx_message','OFF',[]}})  RTISFcnParameters=struct('SFcnRTICANMessage','struct','TLCFileName','char')  RTIBlockParaDefault=struct('BoardTypeNo',4302,'BoardNo',1,'ChannelNo',1,'Parameters',struct('DataFileSupport',struct('DataFileSelectedMaster',0,'DataFileSelectedLocal',0,'DataFileName','','DataFileDate','','SelectedFile',['<no file selected>']),'Options',struct('StatusSelected',1,'TimeSelected',1,'DeltaTimeSelected',1,'BytePortSelected',0,'MessageLengthSelected',0,'TriggerPort',struct('Selected',0,'TriggerType','rising'),'UserCoding',struct('Selected',0,'InterfaceFile','UserDecodingFile','FcnName','UserDecodeFcn','InportSelected',0,'InportWidth',1,'OutportSelected',0,'OutportWidth',1),'EnablePortSelected',0,'SignalOnPortnameSelected',1,'UseRXService',0),'Message',struct('MsgOnBlocknameSelected',0,'MsgName',['RX Message'],'MsgIdFormat',0,'MsgId',100,'MsgLength',8,'NumSignals',1,'SampleTime',-1,'Signal',struct('SgnName',['RX signal'],'SgnStartBit',0,'SgnLength',8,'SgnType',0,'ModeValue',-1,'DataType',0,'SLDataType','SS_DOUBLE','ByteLayout',0,'Factor',1,'Offset',0,'Min',0,'Max',255,'SgnComment',{{}},'SgnUnit',''),'MsgIdNumFormat',0,'MsgComment',{{''}}),'Version',1.2,'general',struct('isFromLib',1)),'GroupId',struct('Group',{{'RTICAN'}},'No',1,'Behavior',{{'NAMECHANGE'}},'BlockType',{{'SINK'}},'NameChangeFlag',0),'SFcnRTICANMessage',struct('MsgType','RX','MsgName',['RX Message'],'MsgIdFormat','STD','MsgId',100,'MsgLength',8,'NumSignals',1,'SampleTime',-1,'Signal',struct('SgnName',['RX signal'],'SgnStartBit',0,'SgnLength',8,'SgnType','standard','ModeValue',-1,'DataType',['unsigned int'],'ByteLayout',['little endian'],'SLDataType','SS_DOUBLE','Factor',1,'Offset',0),'StatusSelected','yes','TimeSelected','yes','DeltaTimeSelected','yes','BytePortSelected','no','MessageLengthSelected','no','EnablePortSelected','no','UserCoding',struct('Selected','no','InterfaceFile','UserDecodingFile','FcnName','UserDecodeFcn','InportSelected','no','InportWidth',1,'OutportSelected','no','OutportWidth',1),'TriggerPort',struct('Selected','no','TriggerType','rising'),'UseRXService','no','BoardType','DS4302','BoardNo',1,'ControllerNo',1,'SFcnPortType','Scalar'),'TLCFileName','rtican_rx_message')
      settings: AttributesFormatString=Group Id: RTICAN4\n
  ESR_Status4_1 : Outport
  wires:
  Bus Creator/1 -> ESR_Status4_1/1  "ESR_Status4"
  ESR_Status4/1 -> Bus Creator/1  "CAN_TX_PATH_ID_ACC_STAT"
  ESR_Status4/2 -> Bus Creator/2  "CAN_TX_AUTO_ALIGN_ANGLE"
  ESR_Status4/3 -> Bus Creator/3  "CAN_TX_PATH_ID_FCW_STAT"
  ESR_Status4/4 -> Bus Creator/4  "CAN_TX_PATH_ID_FCW_MOVE"
  ESR_Status4/5 -> Bus Creator/5  "CAN_TX_PATH_ID_CMBB_STAT"
  ESR_Status4/6 -> Bus Creator/6  "CAN_TX_PATH_ID_CMBB_MOVE"
  ESR_Status4/7 -> Bus Creator/7  "CAN_TX_PATH_ID_ACC"
  ESR_Status4/8 -> Bus Creator/8  "CAN_TX_ROLLING_COUNT_3"
  ESR_Status4/9 -> Bus Creator/9  "CAN_TX_MR_LR_MODE"
  ESR_Status4/10 -> Bus Creator/10  "CAN_TX_PARTIAL_BLOCKAGE"
  ESR_Status4/11 -> Bus Creator/11  "CAN_TX_SIDELOBE_BLOCKAGE"
  ESR_Status4/12 -> Bus Creator/12  "CAN_TX_LR_ONLY_GRATING_LOBE_DET"
  ESR_Status4/13 -> Bus Creator/13  "CAN_TX_TRUCK_TARGET_DET"
